simulink model "svpwm"  (R2019b)
settings: Solver=VariableStepAuto  StartTime=0.0  StopTime=10.0  RelTol=1e-3
settings Model: Creator=srikesh  LastModifiedBy=srikesh

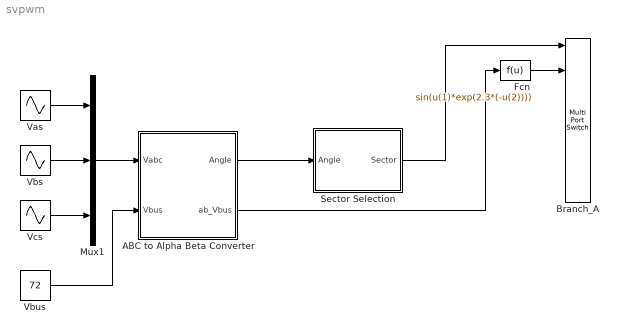
== system svpwm ==
  "ABC to Alpha Beta Converter " : Subsystem
  Branch_A : MultiPortSwitch  Inputs=6  DiagnosticForDefault=None
  Fcn : Fcn  Expr=sin(u(1)*exp(2.3*(-u(2))))
  Mux1 : Mux  Inputs=3
  Sector Selection : Subsystem
  Vas : Sin  Frequency=50  Samples=2*pi/(50*  SampleTime=0
  Vbs : Sin  Frequency=50  Phase=2*pi/3  Samples=2*pi/(50*  SampleTime=0
  Vbus : Constant  Value=72
  Vcs : Sin  Frequency=50  Phase=4*pi/3  Samples=2*pi/(50*  SampleTime=0
  wires:
  Fcn/1 -> Branch_A/2
  Vas/1 -> Mux1/1
  "ABC to Alpha Beta Converter "/1(Angle) -> Sector Selection/1(Angle)
  Vcs/1 -> Mux1/3
  Vbs/1 -> Mux1/2
  Vbus/1 -> "ABC to Alpha Beta Converter "/2(Vbus)
  "ABC to Alpha Beta Converter "/2(ab_Vbus) -> Fcn/1
  Sector Selection/1("Sector ") -> Branch_A/1
  Mux1/1 -> "ABC to Alpha Beta Converter "/1(Vabc)

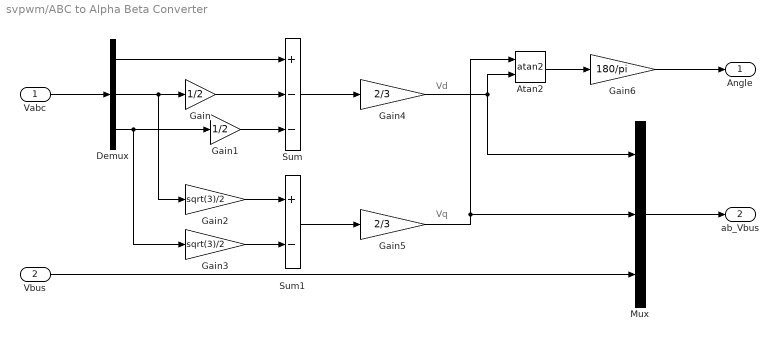
== system svpwm/ABC to Alpha Beta Converter  ==
  note: Vq
  note: Vd
  Vabc : Inport
  Vbus : Inport  Port=2
  Atan2 : Trigonometry  Operator=atan2
  Demux : Demux  Outputs=3
  Gain : Gain  Gain=1/2
  Gain1 : Gain  Gain=1/2
  Gain2 : Gain  Gain=sqrt(3)/2
  Gain3 : Gain  Gain=sqrt(3)/2
  Gain4 : Gain  Gain=2/3
  Gain5 : Gain  Gain=2/3
  Gain6 : Gain  Gain=180/pi
  Mux : Mux  Inputs=3
  Sum : Sum  Inputs=+--
  Sum1 : Sum  Inputs=+-
  Angle : Outport
  ab_Vbus : Outport  Port=2
  wires:
  Vabc/1 -> Demux/1
  Demux/1 -> Sum/1
  Gain/1 -> Sum/2
  Gain1/1 -> Sum/3
  Demux/2 -> Gain2/1, Gain/1
  Demux/3 -> Gain3/1, Gain1/1
  Gain2/1 -> Sum1/1
  Gain3/1 -> Sum1/2
  Sum/1 -> Gain4/1
  Sum1/1 -> Gain5/1
  Gain5/1 -> Atan2/1, Mux/2
  Gain4/1 -> Atan2/2, Mux/1
  Atan2/1 -> Gain6/1
  Gain6/1 -> Angle/1
  Vbus/1 -> Mux/3
  Mux/1 -> ab_Vbus/1

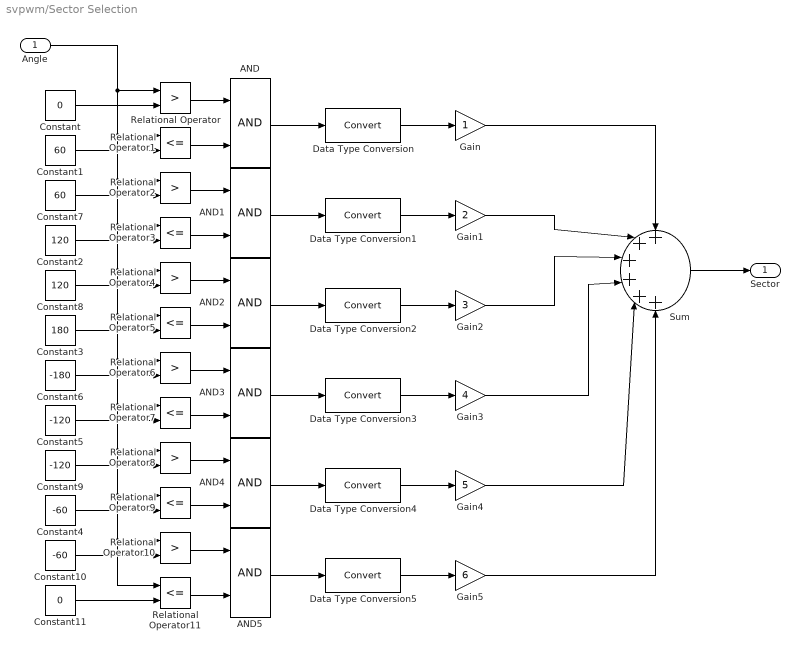
== system svpwm/Sector Selection ==
  Angle : Inport
  AND{,1..5} (6 alike) : Logic  AllPortsSameDT=off  OutDataTypeStr=boolean
  Constant : Constant  Value=0
  Constant1 : Constant  Value=60
  Constant10 : Constant  Value=-60
  Constant11 : Constant  Value=0
  Constant2 : Constant  Value=120
  Constant3 : Constant  Value=180
  Constant4 : Constant  Value=-60
  Constant5 : Constant  Value=-120
  Constant6 : Constant  Value=-180
  Constant7 : Constant  Value=60
  Constant8 : Constant  Value=120
  Constant9 : Constant  Value=-120
  Data Type Conversion{,1..5} (6 alike) : DataTypeConversion
  Gain : Gain
  Gain1 : Gain  Gain=2
  Gain2 : Gain  Gain=3
  Gain3 : Gain  Gain=4
  Gain4 : Gain  Gain=5
  Gain5 : Gain  Gain=6
  Relational Operator{,2,4,6,8,10} (6 alike) : RelationalOperator  Operator=>  OutDataTypeStr=boolean  RndMeth=Simplest
  Relational Operator{1,3,5,7,9,11} (6 alike) : RelationalOperator  Operator=<=  OutDataTypeStr=boolean  RndMeth=Simplest
  Sum : Sum  Inputs=6
  "Sector " : Outport
  wires:
  Constant/1 -> Relational Operator/2
  Constant1/1 -> Relational Operator1/2
  Constant7/1 -> Relational Operator2/2
  Constant2/1 -> Relational Operator3/2
  Constant8/1 -> Relational Operator4/2
  Constant3/1 -> Relational Operator5/2
  Constant6/1 -> Relational Operator6/2
  Constant5/1 -> Relational Operator7/2
  Constant9/1 -> Relational Operator8/2
  Constant4/1 -> Relational Operator9/2
  Constant10/1 -> Relational Operator10/2
  Constant11/1 -> Relational Operator11/2
  Angle/1 -> Relational Operator/1, Relational Operator2/1, Relational Operator5/1, Relational Operator6/1, Relational Operator11/1, Relational Operator10/1, Relational Operator9/1, Relational Operator8/1, Relational Operator7/1, Relational Operator4/1, Relational Operator3/1, Relational Operator1/1
  Relational Operator/1 -> AND/1
  Relational Operator1/1 -> AND/2
  Relational Operator2/1 -> AND1/1
  Relational Operator3/1 -> AND1/2
  Relational Operator4/1 -> AND2/1
  Relational Operator5/1 -> AND2/2
  Relational Operator6/1 -> AND3/1
  Relational Operator7/1 -> AND3/2
  Relational Operator8/1 -> AND4/1
  Relational Operator9/1 -> AND4/2
  Relational Operator10/1 -> AND5/1
  Relational Operator11/1 -> AND5/2
  AND/1 -> Data Type Conversion/1
  AND1/1 -> Data Type Conversion1/1
  AND2/1 -> Data Type Conversion2/1
  AND3/1 -> Data Type Conversion3/1
  AND4/1 -> Data Type Conversion4/1
  AND5/1 -> Data Type Conversion5/1
  Data Type Conversion/1 -> Gain/1
  Data Type Conversion1/1 -> Gain1/1
  Data Type Conversion2/1 -> Gain2/1
  Data Type Conversion3/1 -> Gain3/1
  Data Type Conversion4/1 -> Gain4/1
  Data Type Conversion5/1 -> Gain5/1
  Gain/1 -> Sum/1
  Gain1/1 -> Sum/2
  Gain2/1 -> Sum/3
  Gain3/1 -> Sum/4
  Gain4/1 -> Sum/5
  Sum/1 -> "Sector "/1
  Gain5/1 -> Sum/6
